simulink model "mchp_acim_dsPIC33A"  (R2025b)
settings: Solver=FixedStepDiscrete  StartTime=0.0  StopTime=25  FixedStep=Ts  RelTol=1e-3  EnableMultiTasking=on
values from neighbouring files (symbols this model uses):
  dataType = 'single'    [mchp_acim_foc_dsPIC33A_data.m]
  PWM_frequency = 20e3    (= 20000)    [mchp_acim_foc_dsPIC33A_data.m]
  PWM_frequency_mc = PWM_frequency    (= 20000)    [mchp_acim_foc_dsPIC33A_data.m]
  SpeedFilterCutoff = 40    [mchp_acim_foc_dsPIC33A_data.m]
  Ts = T_pwm    (= 5e-05)    [mchp_acim_foc_dsPIC33A_data.m]
  Ts_mc = T_pwm_mc    (= 5e-05)    [mchp_acim_foc_dsPIC33A_data.m]
  Ts_motor = T_pwm_mc    (= 5e-05)    [mchp_acim_foc_dsPIC33A_data.m]
  Ts_serialIn = 100e-3    (= 0.1)    [mchp_acim_foc_dsPIC33A_data.m]
undefined symbols (not defined in the file or in its folder): A0, A4, acim, ADC, appState, B0, C10, C11, C6, C7, C8, CS_param, D11, D12, DiscIntNeverNeededParam, estim_pll, estim_qei, inverter, Max, MaxPer, ms, NumBits1, NumBits2, P1, P17, P20, P39, P40, P41, P43, P44, P60, P61, PI_params_SI, Pin, PWM4_Trg1, Resol, s, target, us, VmaxPhase
libraries: simulink x47, MCHP_Blockset x24, mcbcontrolslib x5, mcbeeMathTransformLib x4, slpidlib x4, svdutilitieslib x1, autolibim x1, mcbplantlib x1
(part 5 of 6)

== system mchp_acim_dsPIC33A/MCHV-230VAC-1.5kW Development Board dsPIC33AK128MC106 MC DIM/Downsample x20 ==
  note: DownSample & Average by changing data scaling
  In1 : Inport
  Compare To Constant : simulink/Logic and Bit Operations/Compare To Constant  relop===  const=1  OutDataTypeStr=boolean
  Counter Limited : simulink/Sources/Counter Limited  uplimit=DownSample-1  tsamp=-1
  Data Type Duplicate : DataTypeDuplicate
  Data Type Propagation : simulink/Signal Attributes/Data Type Propagation  PropDataType=fixdt(1, 16)  IfRefDouble=double  IfRefSingle=single  IsSigned=IsSigned1 or IsSigned2  NumBitsBase=NumBits1+NumBits2  NumBitsMult=1  NumBitsAdd=0  NumBitsAllowFinal=-1  PropScaling=2^-10  ValuesUsedBestPrec=[5 -7]  SlopeBase=Slope1  SlopeMult=1  SlopeAdd=0  BiasBase=Bias1  BiasMult=1  BiasAdd=0
  Data Type Propagation1 : simulink/Signal Attributes/Data Type Propagation  PropDataType=fixdt(1, 16)  IfRefDouble=double  IfRefSingle=single  IsSigned=IsSigned1 or IsSigned2  NumBitsBase=NumBits1+NumBits2  NumBitsMult=1  NumBitsAdd=0  NumBitsAllowFinal=-1  PropScaling=2^-10  ValuesUsedBestPrec=[5 -7]  SlopeBase=PosRange1  SlopeMult=1  SlopeAdd=0  BiasBase=Bias1  BiasMult=1  BiasAdd=0
  Discrete-Time Integrator : DiscreteIntegrator  IntegratorMethod=Accumulation: Backward Euler  gainval=1  ExternalReset=sampled level  SampleTime=-1  OutDataTypeStr=Inherit: Inherit via back propagation  ICPrevOutput=DiscIntNeverNeededParam  ICPrevScaledInput=DiscIntNeverNeededParam
  Gain : Gain  Gain=1/DownSample  OutDataTypeStr=Inherit: Inherit via back propagation  RndMeth=Round
  Gain1 : Gain  Gain=1/DownSample  OutDataTypeStr=Inherit: Inherit via back propagation
  Rate Transition1 : RateTransition  OutPortSampleTimeOpt=Multiple of input port sample time  OutPortSampleTimeMultiple=DownSample  OutPortSampleTime=DownSample
  Rate Transition3 : RateTransition  OutPortSampleTimeOpt=Multiple of input port sample time  OutPortSampleTimeMultiple=DownSample  OutPortSampleTime=DownSample
  Terminator : Terminator
  Out1 : Outport  VectorParamsAs1DForOutWhenUnconnected=off
  wires:
  Rate Transition3/1 -> Gain1/1, Gain/1
  In1/1 -> Rate Transition1/1, Discrete-Time Integrator/1, Data Type Propagation/2, Data Type Propagation/1
  Compare To Constant/1 -> Discrete-Time Integrator/2
  Discrete-Time Integrator/1 -> Data Type Propagation/3, Rate Transition3/1
  Counter Limited/1 -> Compare To Constant/1
  Gain/1 -> Data Type Duplicate/2, Out1/1
  Rate Transition1/1 -> Data Type Propagation1/2, Data Type Propagation1/1, Data Type Duplicate/1
  Gain1/1 -> Terminator/1, Data Type Propagation1/3

== system mchp_acim_dsPIC33A/MCHV-230VAC-1.5kW Development Board dsPIC33AK128MC106 MC DIM/Downsample x20 _ ==
  note: DownSample & Average by changing data scaling
  In1 : Inport
  Compare To Constant : simulink/Logic and Bit Operations/Compare To Constant  relop===  const=1  OutDataTypeStr=boolean
  Counter Limited : simulink/Sources/Counter Limited  uplimit=DownSample-1  tsamp=-1
  Data Type Duplicate : DataTypeDuplicate
  Data Type Propagation : simulink/Signal Attributes/Data Type Propagation  PropDataType=fixdt(1, 16)  IfRefDouble=double  IfRefSingle=single  IsSigned=IsSigned1 or IsSigned2  NumBitsBase=NumBits1+NumBits2  NumBitsMult=1  NumBitsAdd=0  NumBitsAllowFinal=-1  PropScaling=2^-10  ValuesUsedBestPrec=[5 -7]  SlopeBase=Slope1  SlopeMult=1  SlopeAdd=0  BiasBase=Bias1  BiasMult=1  BiasAdd=0
  Data Type Propagation1 : simulink/Signal Attributes/Data Type Propagation  PropDataType=fixdt(1, 16)  IfRefDouble=double  IfRefSingle=single  IsSigned=IsSigned1 or IsSigned2  NumBitsBase=NumBits1+NumBits2  NumBitsMult=1  NumBitsAdd=0  NumBitsAllowFinal=-1  PropScaling=2^-10  ValuesUsedBestPrec=[5 -7]  SlopeBase=PosRange1  SlopeMult=1  SlopeAdd=0  BiasBase=Bias1  BiasMult=1  BiasAdd=0
  Discrete-Time Integrator : DiscreteIntegrator  IntegratorMethod=Accumulation: Backward Euler  gainval=1  ExternalReset=sampled level  SampleTime=-1  OutDataTypeStr=Inherit: Inherit via back propagation  ICPrevOutput=DiscIntNeverNeededParam  ICPrevScaledInput=DiscIntNeverNeededParam
  Gain : Gain  Gain=1/DownSample  OutDataTypeStr=Inherit: Inherit via back propagation  RndMeth=Round
  Gain1 : Gain  Gain=1/DownSample  OutDataTypeStr=Inherit: Inherit via back propagation
  Rate Transition1 : RateTransition  OutPortSampleTimeOpt=Multiple of input port sample time  OutPortSampleTimeMultiple=DownSample  OutPortSampleTime=DownSample
  Rate Transition3 : RateTransition  OutPortSampleTimeOpt=Multiple of input port sample time  OutPortSampleTimeMultiple=DownSample  OutPortSampleTime=DownSample
  Terminator : Terminator
  Out1 : Outport  VectorParamsAs1DForOutWhenUnconnected=off
  wires:
  Gain1/1 -> Data Type Propagation1/3, Terminator/1
  Rate Transition1/1 -> Data Type Duplicate/1, Data Type Propagation1/1, Data Type Propagation1/2
  Gain/1 -> Out1/1, Data Type Duplicate/2
  Counter Limited/1 -> Compare To Constant/1
  Discrete-Time Integrator/1 -> Rate Transition3/1, Data Type Propagation/3
  Compare To Constant/1 -> Discrete-Time Integrator/2
  In1/1 -> Data Type Propagation/1, Data Type Propagation/2, Discrete-Time Integrator/1, Rate Transition1/1
  Rate Transition3/1 -> Gain/1, Gain1/1

== system mchp_acim_dsPIC33A/MCHV-230VAC-1.5kW Development Board dsPIC33AK128MC106 MC DIM/MCHV-230VAC-1.5kW Development board webpage ==

== system mchp_acim_dsPIC33A/MCHV-230VAC-1.5kW Development Board dsPIC33AK128MC106 MC DIM/Timing Analysis ==
  note: CPU overload is 0 if no overload took place between two MCU Overload block execution.
      | Otherwise, bits field output code for TID(s) responsible for at least one overload.
  Downsample Averaged2 : Subsystem  mask{InputSampleTime=.0005, DownSample=200}
      mask prompts: InputSampleTime "Input sample time"; DownSample "DownSample Factor"
  Gain : Gain  Gain=5e-9/.0005 * 100  OutMin=0  OutMax=100  OutDataTypeStr=fixdt(0,16)  RndMeth=Simplest  SaturateOnIntegerOverflow=on
  MCU Load : MCHP_Blockset/Profiling/MCU Load  MCULoadPin_TXT=None  MCULoadMeasure=on  TIMER_Resolution_TXT="Resol: 0.005(us)  -  Max: 0.328(ms)"  MCHP_TIMER_REQUEST={MCU_Load}{MCU_Load}21:5:0:0:[]:32768;  MCHP_TIMER_RESULT=[2 65535 ]  MCHP_MASTERLINK=mchp_acim_dsPIC33A/MCHV-230VAC-1.5kW Development Board dsPIC33AK128MC106 MC DIM/Microchip Master  MCHP_COMPILED_INFO="CompiledSampleTime= [0.00050000000000000001041   0 ];CompiledInportDataTypes=[    ];CompiledInportDataWidth=[];"  Info="Timer 2:  Resol: 5(ns)  -  Max: 327.68(us)"  SampleTime=.0005
      settings: SourceProductName=MPLAB Device Blocks for Simulink
  MCU Overload : MCHP_Blockset/Profiling/MCU Overload  MCUOverloadBlockOutput=on  MCUOverLoadPin_TXT=None  MCHP_MASTERLINK=mchp_acim_dsPIC33A/MCHV-230VAC-1.5kW Development Board dsPIC33AK128MC106 MC DIM/Microchip Master  SampleTime=-1
      settings: SourceProductName=MPLAB Device Blocks for Simulink
  Overload : Constant  Value=65535  OutDataTypeStr=Inherit: Inherit via back propagation
  Rate Transition : RateTransition  Deterministic=off  OutPortSampleTime=.0005*200
  Switch : Switch  Criteria=u2 ~= 0  SaturateOnIntegerOverflow=off  InputSameDT=off
  CPU Load : Outport  Unit=%  SampleTime=.0005*200
  CPU Overload : Outport  Port=2
  wires:
  Rate Transition/1 -> Switch/2
  MCU Overload/1 -> Rate Transition/1, CPU Overload/1
  MCU Load/1 -> Downsample Averaged2/1(In1)
  Downsample Averaged2/1(Out1) -> Switch/3
  Switch/1 -> Gain/1
  Overload/1 -> Switch/1
  Gain/1 -> CPU Load/1

== system mchp_acim_dsPIC33A/Control algorithm/Application_Abstraction/Subsystem1 ==
  thetaMech_PU : Inport
  Enable : Inport  Port=2
  32-bit PU Angle integrator : Subsystem
  Add : Sum  OutDataTypeStr=single
  Data Type Conversion6 : DataTypeConversion  OutDataTypeStr=fixdt(1,16,15)  RndMeth=Nearest  SaturateOnIntegerOverflow=off
  Data Type Conversion7 : DataTypeConversion  OutDataTypeStr=fixdt(1,16,15)  SaturateOnIntegerOverflow=off  RndMeth=Floor  LockScale=on
  Delay One Step1 : Delay  DelayLength=1  InitialCondition=0  SampleTime=Ts_mc
  Delay One Step5 : Delay  DelayLength=1  InitialCondition=0  ExternalReset=Rising  SampleTime=Ts_mc
      settings: InputPortMap=u0,r5
  Ele_rad/s to mech_rpm : Gain  Gain=60/(2*pi*acim.p)  ParamDataTypeStr=single  OutDataTypeStr=single
  Gain1 : Gain  Gain=(2*estim_qei.zeta_TL/estim_qei.tau_TL)  ParamDataTypeStr=single  OutDataTypeStr=single
  Gain2 : Gain  Gain=Ts_mc*(1/(estim_qei.tau_TL)^2)  OutDataTypeStr=single
  Gain3 : Gain  Gain=acim.p  ParamDataTypeStr=single  OutDataTypeStr=Inherit: Same as input
  LPF : Subsystem
  Subtract5 : Sum  OutDataTypeStr=Inherit: Same as first input
  Sum3 : Sum  Inputs=|+-  OutDataTypeStr=fixdt(1,16,16)
  speed_mech_rpm : Outport
  wires:
  Sum3/1 -> Gain2/1, Gain1/1
  Subtract5/1 -> Delay One Step5/1, Add/1
  Gain2/1 -> Subtract5/1
  Enable/1 -> Delay One Step5/2
  Delay One Step5/1 -> Subtract5/2
  Gain1/1 -> Add/2
  LPF/1(Out) -> speed_mech_rpm/1
  Ele_rad/s to mech_rpm/1 -> LPF/1(In)
  32-bit PU Angle integrator/1(PU_angle_e) -> Delay One Step1/1
  Add/1 -> Ele_rad/s to mech_rpm/1, 32-bit PU Angle integrator/1(speed_ele_rad/s)
  thetaMech_PU/1 -> Data Type Conversion6/1
  Delay One Step1/1 -> Data Type Conversion7/1
  Gain3/1 -> Sum3/1
  Data Type Conversion7/1 -> Sum3/2
  Data Type Conversion6/1 -> Gain3/1

== system mchp_acim_dsPIC33A/Control algorithm/Command_Signals/Triggered Subsystem ==
  Trigger : TriggerPort  TriggerType=falling  VariantControl=Variant
  Delay : Delay  DelayLength=1  InitialCondition=0
  NOT : Logic  Operator=NOT  IconShape=distinctive  AllPortsSameDT=off  OutDataTypeStr=boolean
  RunCmd : Outport
  wires:
  NOT/1 -> RunCmd/1, Delay/1
  Delay/1 -> NOT/1

== system mchp_acim_dsPIC33A/Control algorithm/Data Monitoring/SerialInDrivers ==
  Compare To Constant : simulink/Logic and Bit Operations/Compare To Constant  relop=>=  const=8  OutDataTypeStr=boolean
  Data Type Conversion : DataTypeConversion  SaturateOnIntegerOverflow=off  RndMeth=Floor
  Triggered Subsystem : Subsystem  TreatAsAtomicUnit=on
  UART Rx : MCHP_Blockset/BUS UART/UART Rx  UART_REF=1  Flag_Out=on  Rx_Size_popup=User defined  Rx_Size=8  S_Rx_Size=8  Split=Read all received char  SplitChar=10  OutputDefault_popup=do nothing (end of output vector will be undefined)  OutputDefault=-1  ORDERING=None  SampleTime=Ts_serialIn  MCHP_MASTERLINK=mchp_acim_dsPIC33A/MCHV-230VAC-1.5kW Development Board dsPIC33AK128MC106 MC DIM/Microchip Master  MCHP_COMPILED_INFO="CompiledSampleTime= [0.10000000000000000555   0 ];CompiledInportDataTypes=[    ];CompiledInportDataWidth=[];"
      settings: SourceProductName=MPLAB Device Blocks for Simulink
  SCI_Data : Outport
  wires:
  Compare To Constant/1 -> Triggered Subsystem/Trigger
  UART Rx/1 -> Data Type Conversion/1
  UART Rx/2 -> Triggered Subsystem/1(In1)
  Triggered Subsystem/1(SCI_Data) -> SCI_Data/1
  Data Type Conversion/1 -> Compare To Constant/1

== system mchp_acim_dsPIC33A/Control algorithm/Data Monitoring/SerialOutDrivers ==
  SerialData : Inport
  codegen : Subsystem  VariantControl=(codegen)
  sim : Subsystem  VariantControl=(sim)

== system mchp_acim_dsPIC33A/Control algorithm/Data Monitoring/Subsystem ==
  DebugSel : Inport
  DebugData : Inport  Port=2
  1 : Constant  Value=[1 2]  OutDataTypeStr=uint16  SampleTime=-1
  2 : Constant  Value=[3 4]  OutDataTypeStr=uint16  SampleTime=-1
  3 : Constant  Value=[5 6]  OutDataTypeStr=uint16  SampleTime=-1
  4 : Constant  Value=[7 8]  OutDataTypeStr=uint16  SampleTime=-1
  5 : Constant  Value=[9 10]  OutDataTypeStr=uint16  SampleTime=-1
  6 : Constant  Value=[11 12]  OutDataTypeStr=uint16  SampleTime=-1
  Data_Conditioning_Tx : Subsystem  Variant=on
  Multiport Switch : MultiPortSwitch  Inputs=6  DiagnosticForDefault=None  OutDataTypeStr=uint16  RndMeth=Simplest  SaturateOnIntegerOverflow=off  InputSameDT=off
  Selector : Selector  InputPortWidth=12  IndexOptions=Index vector (port)  Indices=[1 3]  OutputSizes=1
  Debug_signal : Outport
  wires:
  4/1 -> Multiport Switch/5
  DebugData/1 -> Selector/1
  Data_Conditioning_Tx/1(Data_Log) -> Debug_signal/1
  5/1 -> Multiport Switch/6
  1/1 -> Multiport Switch/2
  3/1 -> Multiport Switch/4
  Multiport Switch/1 -> Selector/2
  2/1 -> Multiport Switch/3
  6/1 -> Multiport Switch/7
  Selector/1 -> Data_Conditioning_Tx/1(In1)
  DebugSel/1 -> Multiport Switch/1

== system mchp_acim_dsPIC33A/Control algorithm/Data Monitoring/Variant Subsystem ==
  SCI_Data : Inport
  Mode : Inport  Port=2
  Codegen : Subsystem  VariantControl=(codegen)
  Sim : Subsystem  VariantControl=(sim)
  ConfigAndCommand : Outport
  DebugSel : Outport  Port=2

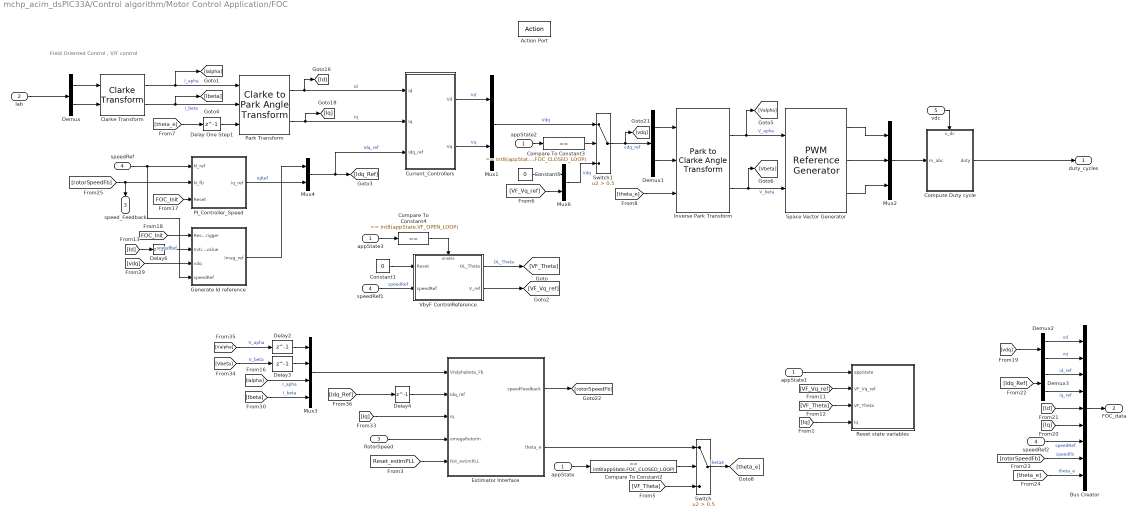
== system mchp_acim_dsPIC33A/Control algorithm/Motor Control Application/FOC ==
  note: Field Oriented Control , V/F control
  appState : Inport
  Iab : Inport  Port=2
  RotorSpeed : Inport  Port=3
  speedRef : Inport  Port=4
  vdc : Inport  Port=5
  Action Port : ActionPort  InitializeStates=reset  PropagateVarSize=During execution  ActionPortLabel=case [ VF_OPEN_LOOP FOC_CLOSED_LOOP ]:
  Bus Creator : BusCreator  Inputs=9
  Clarke Transform : mcbeeMathTransformLib/Clarke Transform  VariantControl=Variant2  PowerInvariant=off  UseWithEmbedded=on  PhaseInput=Two inputs
      settings: LibrarySourceBlock=mcbcontrolslib/Clarke Transform
  Compare To Constant2 : simulink/Logic and Bit Operations/Compare To Constant  relop===  const=int8(appState.FOC_CLOSED_LOOP)  OutDataTypeStr=boolean
  Compare To Constant3 : simulink/Logic and Bit Operations/Compare To Constant  relop===  const=int8(appState.FOC_CLOSED_LOOP)  OutDataTypeStr=boolean
  Compare To Constant4 : simulink/Logic and Bit Operations/Compare To Constant  relop===  const=int8(appState.VF_OPEN_LOOP)  OutDataTypeStr=boolean
  Compute Duty cycle : Subsystem
      settings: PortSchema="{\"entries\":[{\"content\":{\"sides\":[{\"content\":{\"connectorIds\":[\"In1\"]},\"type\":\"ConnectorPlacement.EquallySpacedRectSide\",\"uuid\":\"ac84263d-75b9-49d3-9a57-4d3cc97385b7\"},{\"content\":{\"connectorIds\":[\"Out1\"],\"side\":\"RIGHT\"},\"type\":\"ConnectorPlacement.EquallySpacedRectSide\",\"uuid\":\"0ce133fe-313b-45c1-86d5-76455f259936\"},{\"content\":{\"connectorIds\":[\"In2\"],\"side\":\"TOP\"},\"type\":\"ConnectorPlacement.EquallySpacedRectSide\",\"uuid\":\"39dacd62-df65-4cac-913f-002db890cfc1\"}]},\"type\":\"ConnectorPlacement.EquallySpacedConnector\",\"uuid\":\"58331c50-2548-46fe-a929-f01d574e6535\"}],\"packageUris\":[\"http://schema.mathworks.com/mf0/Connector/R2020b\"],\"version\":\"1.0\"}"
  Constant1 : Constant  Value=0  OutDataTypeStr=single  SampleTime=-1
  Constant5 : Constant  Value=0  OutDataTypeStr=single  SampleTime=-1
  Current_Controllers : Subsystem
  Delay One Step1 : Delay  DelayLength=1
  Delay2 : Delay  DelayLength=1
  Delay3 : Delay  DelayLength=1
  Delay4 : Delay  DelayLength=1  InitialCondition=[0.8, 0.05]
  Delay6 : Delay  DelayLength=1
  Demux{,1..3} (4 alike) : Demux  Outputs=2
  Estimator Interface : Subsystem
  Generate Id reference : Subsystem
  Inverse Park Transform : mcbeeMathTransformLib/Park to Clarke Angle Transform  AxisAlignment=D-axis  UseWithEmbedded=on  PhaseInput=Two inputs  ThetaInput=Electrical position  AngleInput=Radians  N_points=1024
      settings: LibrarySourceBlock=mcbcontrolslib/Inverse Park Transform
  Mux1 : Mux  Inputs=2
  Mux2 : Mux  Inputs=3
  Mux3 : Mux
  Mux4 : Mux  Inputs=2
  Mux6 : Mux  Inputs=2
  PI_Controller_Speed : Subsystem
  Park Transform : mcbeeMathTransformLib/Clarke to Park Angle Transform  AxisAlignment=D-axis  UseWithEmbedded=on  PhaseInput=Two inputs  ThetaInput=Electrical position  AngleInput=Radians  N_points=1024
      settings: LibrarySourceBlock=mcbcontrolslib/Park Transform
  Reset state variables : Subsystem
  Space Vector Generator : mcbcontrolslib/PWM Reference Generator  inSignal=Valphabeta  modType=SVM: space vector modulation
  Switch : Switch  Criteria=u2 > Threshold  Threshold=0.5  SaturateOnIntegerOverflow=off  InputSameDT=off
  Switch1 : Switch  Criteria=u2 > Threshold  Threshold=0.5  SaturateOnIntegerOverflow=off  InputSameDT=off
  VbyF ControlReference : Subsystem
  appState1 : InportShadow
  appState2 : InportShadow
  appState3 : InportShadow
  speedRef1 : InportShadow  Port=4
  speedRef2 : InportShadow  Port=4
  duty_cycles : Outport
  FOC_data : Outport  Port=2
  speed_Feedback : Outport  Port=3
  wires:
  Clarke Transform/2 -> [Ibeta], Park Transform/2  "I_beta"
  Demux/2 -> Clarke Transform/2
  Space Vector Generator/3 -> Mux2/3
  Park Transform/2 -> [Iq], Current_Controllers/2(Iq)  "Iq"
  Park Transform/1 -> [Id], Current_Controllers/1(Id)  "Id"
  Demux/1 -> Clarke Transform/1
  Inverse Park Transform/1 -> Space Vector Generator/1, [Valpha]  "V_apha"
  Clarke Transform/1 -> [Ialpha], Park Transform/1  "I_apha"
  Space Vector Generator/2 -> Mux2/2
  Inverse Park Transform/2 -> Space Vector Generator/2, [Vbeta]  "V_beta"
  Current_Controllers/1(Vd) -> Mux1/1  "Vd"
  Current_Controllers/2(Vq) -> Mux1/2  "Vq"
  Mux1/1 -> Switch1/1  "Vdq"
  Iab/1 -> Demux/1
  Bus Creator/1 -> FOC_data/1
  Demux1/1 -> Inverse Park Transform/1
  Demux1/2 -> Inverse Park Transform/2
  VbyF ControlReference/2(V_ref) -> [VF_Vq_ref]
  speedRef/1 -> Generate Id reference/4(speedRef), PI_Controller_Speed/1(N_ref)  "speedRef"
  VbyF ControlReference/1(OL_Theta) -> [VF_Theta]  "OL_Theta"
  Constant1/1 -> VbyF ControlReference/1(Reset)
  Generate Id reference/1(Imag_ref) -> Mux4/1
  PI_Controller_Speed/1(Iq_ref) -> Mux4/2  "IqRef"
  Mux4/1 -> [Idq_Ref], Current_Controllers/3(Idq_ref)  "Idq_ref"
  appState/1 -> Compare To Constant2/1
  [VF_Theta] -> Switch/3
  Compare To Constant2/1 -> Switch/2
  [VF_Vq_ref] -> Mux6/2
  Constant5/1 -> Mux6/1
  appState2/1 -> Compare To Constant3/1
  Compare To Constant3/1 -> Switch1/2
  Mux6/1 -> Switch1/3  "Vdq"
  Switch1/1 -> Demux1/1, [vdq]  "vdq_ref"
  [theta_e] -> Delay One Step1/1
  [theta_e] -> Inverse Park Transform/3
  speedRef1/1 -> VbyF ControlReference/2(speedRef)  "speedRef"
  [Id] -> Delay6/1
  Delay6/1 -> Generate Id reference/2(Initial_value)
  Space Vector Generator/1 -> Mux2/1
  [FOC_Init] -> PI_Controller_Speed/3(Reset)
  [FOC_Init] -> Generate Id reference/1(Reset_trigger)
  [vdq] -> Demux2/1
  [Idq_Ref] -> Demux3/1
  [Id] -> Bus Creator/5
  [Iq] -> Bus Creator/6
  [rotorSpeedFb] -> Bus Creator/8  "speedFb"
  [theta_e] -> Bus Creator/9  "theta_e"
  speedRef2/1 -> Bus Creator/7  "speedRef"
  [rotorSpeedFb] -> PI_Controller_Speed/2(N_fb), speed_Feedback/1
  Mux2/1 -> Compute Duty cycle/1(m_abc)
  Compute Duty cycle/1(duty) -> duty_cycles/1
  vdc/1 -> Compute Duty cycle/2(v_dc)
  [vdq] -> Generate Id reference/3(vdq)
  appState1/1 -> Reset state variables/1(appState)
  appState3/1 -> Compare To Constant4/1
  Compare To Constant4/1 -> VbyF ControlReference/Enable
  Mux3/1 -> Estimator Interface/1(VIalphabeta_Fb)
  [Idq_Ref] -> Delay4/1
  [Valpha] -> Delay2/1  "V_apha"
  Delay2/1 -> Mux3/1
  Delay4/1 -> Estimator Interface/2(Idq_ref)
  [Ibeta] -> Mux3/4  "I_beta"
  [Vbeta] -> Delay3/1  "V_beta"
  Delay3/1 -> Mux3/2
  [Ialpha] -> Mux3/3  "I_apha"
  [Iq] -> Estimator Interface/3(Iq)
  RotorSpeed/1 -> Estimator Interface/4(omegaRotorIn)
  Estimator Interface/1(speedFeedback) -> [rotorSpeedFb]
  Estimator Interface/2(theta_e) -> Switch/1
  Delay One Step1/1 -> Park Transform/3
  Switch/1 -> [theta_e]  "thetaE"
  [VF_Vq_ref] -> Reset state variables/2(VF_Vq_ref)
  [VF_Theta] -> Reset state variables/3(VF_Theta)
  [Iq] -> Reset state variables/4(Iq)
  Demux3/2 -> Bus Creator/4  "iq_ref"
  Demux3/1 -> Bus Creator/3  "id_ref"
  Demux2/2 -> Bus Creator/2  "vq"
  Demux2/1 -> Bus Creator/1  "vd"
  [Reset_estimPLL] -> Estimator Interface/5(Rst_estimPLL)

== system mchp_acim_dsPIC33A/Control algorithm/Motor Control Application/Switch Case Action Subsystem ==
  Action Port : ActionPort  ActionPortLabel=case [ INIT ]:
  Constant10 : Constant  Value=[0 0 0]  OutDataTypeStr=dataType  SampleTime=Ts_mc
  Duty_Cycles : Outport
  wires:
  Constant10/1 -> Duty_Cycles/1

== system mchp_acim_dsPIC33A/Control algorithm/Motor Control Application/Switch Case Action Subsystem1 ==
  Action Port : ActionPort  ActionPortLabel=case [ OFFSET_MEAS ]:
  Constant10 : Constant  Value=[0 0 0]  OutDataTypeStr=dataType  SampleTime=Ts_mc
  Duty_Cycles : Outport
  wires:
  Constant10/1 -> Duty_Cycles/1

== system mchp_acim_dsPIC33A/Control algorithm/Motor Control Application/Switch Case Action Subsystem6 ==
  Action Port : ActionPort  ActionPortLabel=case [ CMD_WAIT ]:
  Constant10 : Constant  Value=[0 0 0]  OutDataTypeStr=dataType  SampleTime=Ts_mc
  Duty_Cycles : Outport
  wires:
  Constant10/1 -> Duty_Cycles/1

== system mchp_acim_dsPIC33A/Control algorithm/Motor Control Application/Switch Case Action Subsystem8 ==
  Action Port : ActionPort  ActionPortLabel=case [ STOP ]:
  Constant10 : Constant  Value=[0 0 0]  OutDataTypeStr=dataType  SampleTime=Ts_mc
  Duty_Cycles : Outport
  wires:
  Constant10/1 -> Duty_Cycles/1

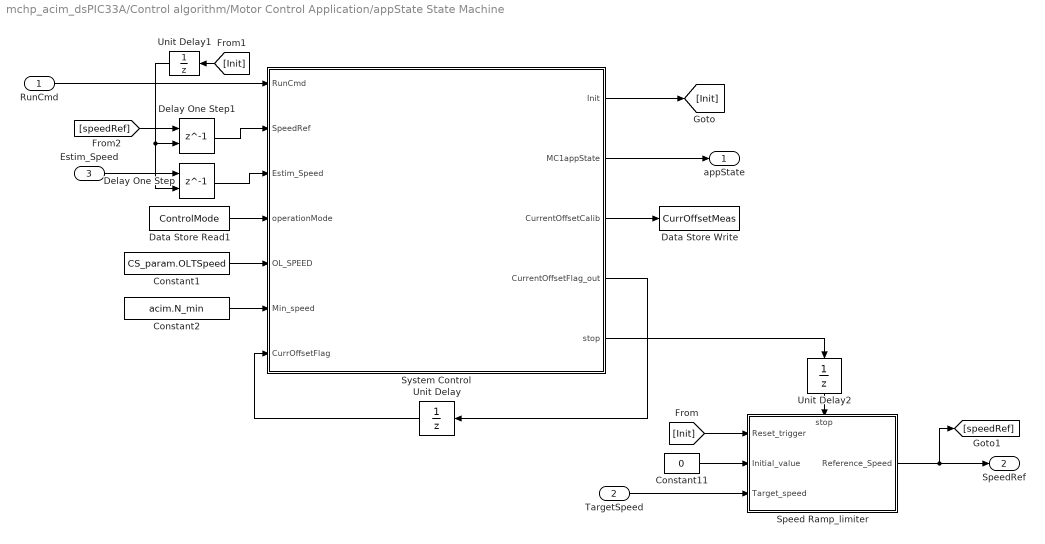
== system mchp_acim_dsPIC33A/Control algorithm/Motor Control Application/appState State Machine ==
  RunCmd : Inport
  TargetSpeed : Inport  Port=2
  Estim_Speed : Inport  Port=3
  Constant1 : Constant  Value=CS_param.OLTSpeed  OutDataTypeStr=single  SampleTime=-1
  Constant11 : Constant  Value=0  OutDataTypeStr=single  SampleTime=-1
  Constant2 : Constant  Value=acim.N_min  OutDataTypeStr=single  SampleTime=-1
  Data Store Read1 : DataStoreRead  DataStoreName=ControlMode  IndexOptions=Index vector (dialog)  Indices=1  OutputSizes=1
  Data Store Write : DataStoreWrite  DataStoreName=CurrOffsetMeas  IndexOptions=Index vector (dialog)  Indices=1  OutputSizes=1
  Delay One Step : Delay  DelayLength=1  ExternalReset=Rising
      settings: InputPortMap=u0,r5
  Delay One Step1 : Delay  DelayLength=1  ExternalReset=Rising
      settings: InputPortMap=u0,r5
  Speed Ramp_limiter : Subsystem
      settings: PortSchema="{\"entries\":[{\"content\":{\"sides\":[{\"content\":{\"connectorIds\":[\"In1\",\"In2\",\"In3\"]},\"type\":\"ConnectorPlacement.EquallySpacedRectSide\",\"uuid\":\"e8ad02be-694d-4221-8646-4c084b3944db\"},{\"content\":{\"connectorIds\":[\"Out1\"],\"side\":\"RIGHT\"},\"type\":\"ConnectorPlacement.EquallySpacedRectSide\",\"uuid\":\"a085ae95-de52-4e1d-a5b3-22bb50ad6f9b\"},{\"content\":{\"connectorIds\":[\"In4\"],\"side\":\"TOP\"},\"type\":\"ConnectorPlacement.EquallySpacedRectSide\",\"uuid\":\"9578737c-df7e-4f95-9460-5c8a62b1220e\"}]},\"type\":\"ConnectorPlacement.EquallySpacedConnector\",\"uuid\":\"d1810837-ee07-43de-beea-054fa145336d\"}],\"packageUris\":[\"http://schema.mathworks.com/mf0/Connector/R2020b\"],\"version\":\"1.0\"}"
  System Control : Stateflow chart  TreatAsAtomicUnit=on
      settings: PortSchema="{\"entries\":[{\"content\":{\"sides\":[{\"content\":{\"connectorIds\":[\"In1\",\"In2\",\"In5\",\"In3\",\"In4\",\"In6\",\"In7\"]},\"type\":\"ConnectorPlacement.EquallySpacedRectSide\",\"uuid\":\"55763e8d-7f73-4f84-bcf2-4b2b0f0a00bd\"},{\"content\":{\"connectorIds\":[\"Out2\",\"Out1\",\"Out3\",\"Out4\",\"Out5\"],\"side\":\"RIGHT\"},\"type\":\"ConnectorPlacement.EquallySpacedRectSide\",\"uuid\":\"fa80ef7b-287b-433f-8260-ff03a517800f\"},{\"content\":{\"side\":\"TOP\"},\"type\":\"ConnectorPlacement.EquallySpacedRectSide\",\"uuid\":\"8900c884-cbcc-4066-bc5f-6440d28e0400\"}]},\"type\":\"ConnectorPlacement.EquallySpacedConnector\",\"uuid\":\"d1ec0316-c890-471e-a041-a7780a4a6b79\"}],\"packageUris\":[\"http://schema.mathworks.com/mf0/Connector/R2020b\"],\"version\":\"1.0\"}"
  Unit Delay : UnitDelay  SampleTime=Ts_mc  HasFrameUpgradeWarning=on
  Unit Delay1 : UnitDelay  SampleTime=Ts_mc  HasFrameUpgradeWarning=on
  Unit Delay2 : UnitDelay  SampleTime=Ts_mc  HasFrameUpgradeWarning=on
  appState : Outport
  SpeedRef : Outport  Port=2
  wires:
  System Control/1(MC1appState) -> appState/1
  RunCmd/1 -> System Control/1(RunCmd)
  System Control/3(CurrentOffsetCalib) -> Data Store Write/1
  Speed Ramp_limiter/1(Reference_Speed) -> SpeedRef/1, [speedRef]
  System Control/4(CurrentOffsetFlag_out) -> Unit Delay/1
  Unit Delay/1 -> System Control/7(CurrOffsetFlag)
  Estim_Speed/1 -> Delay One Step/1
  Constant1/1 -> System Control/4(OL_SPEED)
  Delay One Step/1 -> System Control/5(Estim_Speed)
  Delay One Step1/1 -> System Control/2(SpeedRef)
  Unit Delay1/1 -> Delay One Step/2, Delay One Step1/2
  System Control/2(Init) -> [Init]
  Constant11/1 -> Speed Ramp_limiter/2(Initial_value)
  TargetSpeed/1 -> Speed Ramp_limiter/3(Target_speed)
  System Control/5(stop) -> Unit Delay2/1
  Unit Delay2/1 -> Speed Ramp_limiter/4(stop)
  Data Store Read1/1 -> System Control/3(operationMode)
  [Init] -> Unit Delay1/1
  [Init] -> Speed Ramp_limiter/1(Reset_trigger)
  [speedRef] -> Delay One Step1/1
  Constant2/1 -> System Control/6(Min_speed)

== system mchp_acim_dsPIC33A/Inverter and Motor model/Simulation/Load_Profile (Torque) ==
  Data Type Conversion : DataTypeConversion  OutDataTypeStr=single  SaturateOnIntegerOverflow=off  RndMeth=Floor
  IIR Filter : mcbcontrolslib/IIR Filter  VariantControl=Low Pass Filter  VariantSelect=Low-pass  FilterConstantInputType=Specify via dialog  Filter_constant=0.01  InitialOutput=Specify via dialog  InitialOutputValue=0  ExternalReset=none  advancedSettings=off  Ts=50e-6  cutOff_freq=32.1525
  Reversal : Step  Time=9
  Switch : Switch  Criteria=u2 > Threshold  SaturateOnIntegerOverflow=off  InputSameDT=off
  T_load : Step  Time=3  Before=0.05*acim.T_rated  After=0.3*acim.T_rated  SampleTime=Ts
  T_load1 : Step  Time=6  Before=0.3*acim.T_rated  After=-0.3*acim.T_rated  SampleTime=Ts
  Load_Trq : Outport  VectorParamsAs1DForOutWhenUnconnected=off
  wires:
  Switch/1 -> Data Type Conversion/1
  Data Type Conversion/1 -> IIR Filter/1
  IIR Filter/1 -> Load_Trq/1
  T_load1/1 -> Switch/1
  Reversal/1 -> Switch/2
  T_load/1 -> Switch/3

== system mchp_acim_dsPIC33A/Inverter and Motor model/Simulation/Motor and Inverter ==
  Vabc_In_PU : Inport
  Load : Inport  Port=2
  Bus Selector : BusSelector  OutputSignals=MtrMechPos
  Induction Motor : autolibim/Induction Motor  sim_type=Discrete  Ts=Ts_motor  port_config=Torque  P=acim.p  Zs=[acim.Rs, acim.Lls]  Zr=[acim.Rr, acim.Llr]  Lm=acim.Lm  mechanical=[acim.J, acim.B, 0]  theta_init=0  omega_init=0  RefBlkName='autolibim/Induction Motor'  aMode=5
      settings: LibrarySourceBlock=mcblib/Electrical Systems/Motors/Induction Motor
  Inverter : Subsystem
  RT1 : RateTransition  Deterministic=off  OutPortSampleTime=Ts_simulink
  RT3 : RateTransition  Deterministic=off  OutPortSampleTime=Ts_simulink
  Rate Transition : RateTransition  Integrity=off  OutPortSampleTime=Ts_motor
  Rate Transition1 : RateTransition  Integrity=off  OutPortSampleTime=Ts_motor
  Rate Transition2 : RateTransition  Deterministic=off  OutPortSampleTime=Ts
  Rate Transition3 : RateTransition  Deterministic=off  OutPortSampleTime=Ts
  Scope : Scope
      settings: ActiveDisplayYMinimum=-1  ActiveDisplayYMaximum=1  DataLoggingVariableName=ScopeData4
  Scope1 : Scope  NumInputPorts=2
      settings: ActiveDisplayYMinimum=-142.50303268432617  ActiveDisplayYMaximum=142.50303268432617  DataLoggingVariableName=ScopeData6
  Terminator1 : Terminator
  Iabc : Outport
  Theta : Outport  Port=2
  wires:
  Rate Transition3/1 -> Inverter/1(Duty_abc)
  Rate Transition2/1 -> Rate Transition1/1
  Bus Selector/1 -> Theta/1  "<MtrMechPos>"
  RT3/1 -> Bus Selector/1
  RT1/1 -> Iabc/1
  Vabc_In_PU/1 -> Rate Transition3/1
  Inverter/1(Vabc) -> Rate Transition/1
  Rate Transition1/1 -> Induction Motor/1
  Induction Motor/2 -> Scope1/2, RT1/1  "Iabc_motor"
  Rate Transition/1 -> Scope1/1, Induction Motor/2  "Vabc_motor"
  Load/1 -> Rate Transition2/1
  Induction Motor/1 -> RT3/1
  Induction Motor/3 -> Scope/1, Terminator1/1  "speed_plant_motor"

== system mchp_acim_dsPIC33A/Inverter and Motor model/Simulation/Sensor_Measurements ==
  note: Scaling
  note: Delays
  PhaseCurr : Inport
  pos : Inport  Port=2
  Bus Creator : BusCreator  Inputs=2
  Data Type Conversion2 : DataTypeConversion  OutDataTypeStr=single  RndMeth=Simplest  SaturateOnIntegerOverflow=off
  Data Type Conversion4 : DataTypeConversion  OutDataTypeStr=single  RndMeth=Simplest  SaturateOnIntegerOverflow=off
  Data Type Conversion7 : DataTypeConversion  OutDataTypeStr=single  RndMeth=Simplest  SaturateOnIntegerOverflow=off
  Delay1 : Delay  DelayLength=PI_params_SI.delay_Currents
  Delay2 : Delay  DelayLength=PI_params_SI.delay_Position
  Get_QEP_Counts : Gain  Gain=acim.QEPSlits*4/(2*pi)  OutDataTypeStr=int32  RndMeth=Simplest
  Selector : Selector  InputPortWidth=3  IndexOptions=Index vector (dialog)  Indices=[1 2]  OutputSizes=1
  Sim_fb : Outport  VectorParamsAs1DForOutWhenUnconnected=off
  wires:
  Delay1/1 -> Selector/1  "Iab_fb"
  Data Type Conversion4/1 -> Delay1/1
  Selector/1 -> Bus Creator/1  "Iab_plant_model"
  PhaseCurr/1 -> Data Type Conversion4/1
  Bus Creator/1 -> Sim_fb/1
  Data Type Conversion2/1 -> Delay2/1  "Theta_m_motor"
  Delay2/1 -> Get_QEP_Counts/1  "Theta_m"
  Get_QEP_Counts/1 -> Data Type Conversion7/1  "Theta_qep"
  pos/1 -> Data Type Conversion2/1
  Data Type Conversion7/1 -> Bus Creator/2  "position_count"

== system mchp_acim_dsPIC33A/MCHV-230VAC-1.5kW Development Board dsPIC33AK128MC106 MC DIM/Center & sign reversal/Downsample Averaged 2000 samples remove bias ==
  note: DownSample & Average by changing data scaling
  In1 : Inport
  Enable : EnablePort
  Compare To Constant : simulink/Logic and Bit Operations/Compare To Constant  relop===  const=1  OutDataTypeStr=boolean
  Counter Limited : simulink/Sources/Counter Limited  uplimit=DownSample-1  tsamp=-1
  Data Type Duplicate : DataTypeDuplicate
  Data Type Propagation : simulink/Signal Attributes/Data Type Propagation  PropDataType=fixdt(1, 16)  IfRefDouble=double  IfRefSingle=single  IsSigned=IsSigned1 or IsSigned2  NumBitsBase=NumBits1+NumBits2  NumBitsMult=1  NumBitsAdd=0  NumBitsAllowFinal=-1  PropScaling=2^-10  ValuesUsedBestPrec=[5 -7]  SlopeBase=Slope1  SlopeMult=1  SlopeAdd=0  BiasBase=Bias1  BiasMult=1  BiasAdd=0
  Data Type Propagation1 : simulink/Signal Attributes/Data Type Propagation  PropDataType=fixdt(1, 16)  IfRefDouble=double  IfRefSingle=single  IsSigned=IsSigned1 or IsSigned2  NumBitsBase=NumBits1+NumBits2  NumBitsMult=1  NumBitsAdd=0  NumBitsAllowFinal=-1  PropScaling=2^-10  ValuesUsedBestPrec=[5 -7]  SlopeBase=PosRange1  SlopeMult=1  SlopeAdd=0  BiasBase=Bias1  BiasMult=1  BiasAdd=0
  Discrete-Time Integrator : DiscreteIntegrator  IntegratorMethod=Accumulation: Backward Euler  gainval=1  ExternalReset=sampled level  SampleTime=-1  OutDataTypeStr=Inherit: Inherit via back propagation  ICPrevOutput=DiscIntNeverNeededParam  ICPrevScaledInput=DiscIntNeverNeededParam
  Gain : Gain  Gain=1/DownSample  OutDataTypeStr=uint16  RndMeth=Round
  Gain1 : Gain  Gain=1/DownSample  OutDataTypeStr=Inherit: Inherit via back propagation
  Gain2 : Gain  OutDataTypeStr=int32
  Rate Transition1 : RateTransition  OutPortSampleTimeOpt=Multiple of input port sample time  OutPortSampleTimeMultiple=DownSample  OutPortSampleTime=DownSample
  Rate Transition3 : RateTransition  OutPortSampleTimeOpt=Multiple of input port sample time  OutPortSampleTimeMultiple=DownSample  OutPortSampleTime=DownSample
  Terminator : Terminator
  Out1 : Outport  InitialOutput=[32768]  VectorParamsAs1DForOutWhenUnconnected=off
  wires:
  Gain1/1 -> Gain2/1, Data Type Propagation1/3  "Offset"
  Rate Transition1/1 -> Data Type Duplicate/1, Data Type Propagation1/1, Data Type Propagation1/2
  Gain/1 -> Terminator/1, Data Type Duplicate/2  "Offset_Value_Uint16"
  Counter Limited/1 -> Compare To Constant/1
  Discrete-Time Integrator/1 -> Rate Transition3/1, Data Type Propagation/3  "Intergrator_Out"
  Compare To Constant/1 -> Discrete-Time Integrator/2
  In1/1 -> Data Type Propagation/1, Data Type Propagation/2, Discrete-Time Integrator/1, Rate Transition1/1
  Rate Transition3/1 -> Gain/1, Gain1/1
  Gain2/1 -> Out1/1  "Offset_Value_int32"

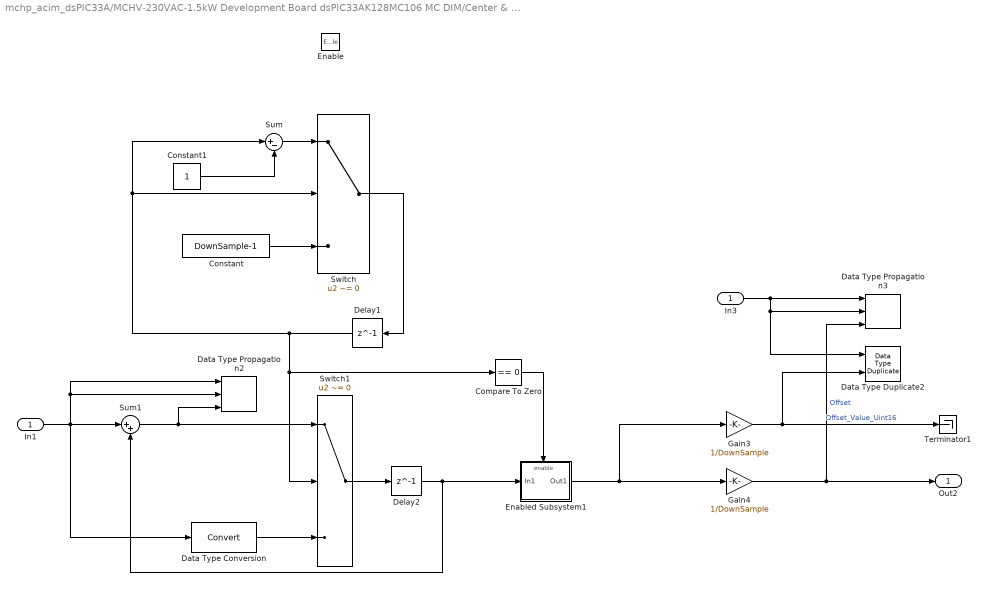
== system mchp_acim_dsPIC33A/MCHV-230VAC-1.5kW Development Board dsPIC33AK128MC106 MC DIM/Center & sign reversal1/Moving Average ==
  In1 : Inport
  Enable : EnablePort  ZeroCross=off
  Compare To Zero : simulink/Logic and Bit Operations/Compare To Zero  relop===  OutDataTypeStr=boolean
  Constant : Constant  Value=DownSample-1  OutDataTypeStr=uint16
  Constant1 : Constant  OutDataTypeStr=uint16
  Data Type Duplicate2 : DataTypeDuplicate
  Data Type Propagation2 : simulink/Signal Attributes/Data Type Propagation  PropDataType=fixdt(1, 16)  IfRefDouble=double  IfRefSingle=single  IsSigned=IsSigned1 or IsSigned2  NumBitsBase=NumBits1+NumBits2  NumBitsMult=1  NumBitsAdd=0  NumBitsAllowFinal=-1  PropScaling=2^-10  ValuesUsedBestPrec=[5 -7]  SlopeBase=Slope1  SlopeMult=1  SlopeAdd=0  BiasBase=Bias1  BiasMult=1  BiasAdd=0
  Data Type Propagation3 : simulink/Signal Attributes/Data Type Propagation  PropDataType=fixdt(1, 16)  IfRefDouble=double  IfRefSingle=single  IsSigned=IsSigned1 or IsSigned2  NumBitsBase=NumBits1+NumBits2  NumBitsMult=1  NumBitsAdd=0  NumBitsAllowFinal=-1  PropScaling=2^-10  ValuesUsedBestPrec=[5 -7]  SlopeBase=PosRange1  SlopeMult=1  SlopeAdd=0  BiasBase=Bias1  BiasMult=1  BiasAdd=0
  Data Type Conversion : DataTypeConversion  SaturateOnIntegerOverflow=off  RndMeth=Floor
  Delay1 : Delay  DelayLength=1  InitialCondition=0
  Delay2 : Delay  DelayLength=1  InitialCondition=[InitialValue * DownSample]
  Enabled Subsystem1 : Subsystem  TreatAsAtomicUnit=on
  Gain3 : Gain  Gain=1/DownSample  OutDataTypeStr=Inherit: Inherit via back propagation  RndMeth=Round
  Gain4 : Gain  Gain=1/DownSample  OutDataTypeStr=Inherit: Inherit via back propagation
  In3 : InportShadow
  Sum : Sum  Inputs=|+-  InputSameDT=on  OutDataTypeStr=Inherit: Same as first input
  Sum1 : Sum  Inputs=|++
  Switch : Switch  Criteria=u2 ~= 0  Threshold=DownSample-1  SaturateOnIntegerOverflow=off  InputSameDT=off
  Switch1 : Switch  Criteria=u2 ~= 0  Threshold=DownSample-1  SaturateOnIntegerOverflow=off
  Terminator1 : Terminator
  Out2 : Outport  InitialOutput=[InitialValue]  VectorParamsAs1DForOutWhenUnconnected=off
  wires:
  Switch/1 -> Delay1/1
  Sum/1 -> Switch/1
  Constant1/1 -> Sum/2
  Constant/1 -> Switch/3
  Delay1/1 -> Switch/2, Sum/1, Switch1/2, Compare To Zero/1
  Delay2/1 -> Sum1/2, Enabled Subsystem1/1(In1)
  In1/1 -> Data Type Conversion/1, Data Type Propagation2/2, Data Type Propagation2/1, Sum1/1
  Sum1/1 -> Data Type Propagation2/3, Switch1/1
  Switch1/1 -> Delay2/1
  Compare To Zero/1 -> Enabled Subsystem1/Enable
  Gain3/1 -> Data Type Duplicate2/2, Terminator1/1  "Offset_Value_Uint16"
  Enabled Subsystem1/1(Out1) -> Gain4/1, Gain3/1
  Gain4/1 -> Out2/1, Data Type Propagation3/3  "Offset"
  In3/1 -> Data Type Duplicate2/1, Data Type Propagation3/2, Data Type Propagation3/1
  Data Type Conversion/1 -> Switch1/3

== system mchp_acim_dsPIC33A/MCHV-230VAC-1.5kW Development Board dsPIC33AK128MC106 MC DIM/Timing Analysis/Downsample Averaged2 ==
  note: DownSample & Average by changing data scaling
  In1 : Inport
  Compare To Constant : simulink/Logic and Bit Operations/Compare To Constant  relop===  const=1  OutDataTypeStr=boolean
  Counter Limited : simulink/Sources/Counter Limited  uplimit=DownSample-1  tsamp=-1
  Data Type Duplicate : DataTypeDuplicate
  Data Type Propagation : simulink/Signal Attributes/Data Type Propagation  PropDataType=fixdt(1, 16)  IfRefDouble=double  IfRefSingle=single  IsSigned=IsSigned1 or IsSigned2  NumBitsBase=NumBits1+NumBits2  NumBitsMult=1  NumBitsAdd=0  NumBitsAllowFinal=-1  PropScaling=2^-10  ValuesUsedBestPrec=[5 -7]  SlopeBase=Slope1  SlopeMult=1  SlopeAdd=0  BiasBase=Bias1  BiasMult=1  BiasAdd=0
  Data Type Propagation1 : simulink/Signal Attributes/Data Type Propagation  PropDataType=fixdt(1, 16)  IfRefDouble=double  IfRefSingle=single  IsSigned=IsSigned1 or IsSigned2  NumBitsBase=NumBits1+NumBits2  NumBitsMult=1  NumBitsAdd=0  NumBitsAllowFinal=-1  PropScaling=2^-10  ValuesUsedBestPrec=[5 -7]  SlopeBase=PosRange1  SlopeMult=1  SlopeAdd=0  BiasBase=Bias1  BiasMult=1  BiasAdd=0
  Discrete-Time Integrator : DiscreteIntegrator  IntegratorMethod=Accumulation: Backward Euler  gainval=1  ExternalReset=sampled level  SampleTime=-1  OutDataTypeStr=Inherit: Inherit via back propagation  ICPrevOutput=DiscIntNeverNeededParam  ICPrevScaledInput=DiscIntNeverNeededParam
  Gain : Gain  Gain=1/DownSample  OutDataTypeStr=Inherit: Inherit via back propagation
  Gain1 : Gain  Gain=1/DownSample  OutDataTypeStr=Inherit: Inherit via back propagation
  Rate Transition1 : RateTransition  Deterministic=off  OutPortSampleTime=[InputSampleTime * DownSample]
  Rate Transition3 : RateTransition  OutPortSampleTime=[InputSampleTime * DownSample]
  Terminator : Terminator
  Out1 : Outport  VectorParamsAs1DForOutWhenUnconnected=off
  wires:
  Rate Transition3/1 -> Gain1/1, Gain/1
  In1/1 -> Discrete-Time Integrator/1, Rate Transition1/1, Data Type Propagation/2, Data Type Propagation/1
  Compare To Constant/1 -> Discrete-Time Integrator/2
  Discrete-Time Integrator/1 -> Data Type Propagation/3, Rate Transition3/1
  Counter Limited/1 -> Compare To Constant/1
  Gain/1 -> Data Type Duplicate/2, Out1/1
  Rate Transition1/1 -> Data Type Propagation1/2, Data Type Propagation1/1, Data Type Duplicate/1
  Gain1/1 -> Data Type Propagation1/3, Terminator/1

== system mchp_acim_dsPIC33A/Control algorithm/Application_Abstraction/Subsystem1/32-bit PU Angle integrator ==
  speed_ele_rad/s : Inport
  " " : Gain  Gain=Ts_mc  ParamDataTypeStr=single  OutDataTypeStr=single
  Data Type Conversion1 : DataTypeConversion  OutDataTypeStr=fixdt(1,32,31)  SaturateOnIntegerOverflow=off  RndMeth=Floor
  Data Type Conversion3 : DataTypeConversion  OutDataTypeStr=fixdt(1,16,15)  SaturateOnIntegerOverflow=off  RndMeth=Floor
  Delay One Step1 : Delay  DelayLength=1  InitialCondition=0  SampleTime=Ts_mc
  PU : Gain  Gain=1/pi  ParamDataTypeStr=single  OutDataTypeStr=single
  Subtract1 : Sum  OutDataTypeStr=fixdt(1,32,31)
  PU_angle_e : Outport
  wires:
  PU/1 -> Data Type Conversion1/1
  " "/1 -> PU/1
  Delay One Step1/1 -> Subtract1/2
  Data Type Conversion1/1 -> Subtract1/1
  Subtract1/1 -> Data Type Conversion3/1, Delay One Step1/1
  Data Type Conversion3/1 -> PU_angle_e/1
  speed_ele_rad/s/1 -> " "/1

== system mchp_acim_dsPIC33A/Control algorithm/Application_Abstraction/Subsystem1/LPF ==
  In : Inport
  Delay One Step : Delay  DelayLength=1  SampleTime=Ts_mc
  Gain : Gain  Gain=Ts_mc/((1/(2*pi*SpeedFilterCutoff))+Ts_mc)  ParamDataTypeStr=single  OutDataTypeStr=single
  Subtract : Sum  Inputs=+-
  Subtract1 : Sum  OutDataTypeStr=Inherit: Inherit via back propagation
  Out : Outport
  wires:
  In/1 -> Subtract/1
  Subtract1/1 -> Delay One Step/1, Out/1
  Delay One Step/1 -> Subtract1/2, Subtract/2
  Subtract/1 -> Gain/1
  Gain/1 -> Subtract1/1

== system mchp_acim_dsPIC33A/Control algorithm/Data Monitoring/SerialInDrivers/Triggered Subsystem ==
  In1 : Inport
  Trigger : TriggerPort  VariantControl=(inherit)
  SCI_Data : Outport
  wires:
  In1/1 -> SCI_Data/1

== system mchp_acim_dsPIC33A/Control algorithm/Data Monitoring/SerialOutDrivers/codegen ==
  SerialData : Inport
  SCI_Tx : Subsystem
  wires:
  SerialData/1 -> SCI_Tx/1(Data_Log)

== system mchp_acim_dsPIC33A/Control algorithm/Data Monitoring/SerialOutDrivers/sim ==
  SerialData : Inport
  Terminator : Terminator
  wires:
  SerialData/1 -> Terminator/1

== system mchp_acim_dsPIC33A/Control algorithm/Data Monitoring/Subsystem/Data_Conditioning_Tx ==
  In1 : Inport
  Data_Type_Fixed_Point : Subsystem  VariantControl=~isequal(dataType,'single')
  Data_Type_Float : Subsystem  VariantControl=isequal(dataType, 'single')
  Data_Log : Outport

== system mchp_acim_dsPIC33A/Control algorithm/Data Monitoring/Variant Subsystem/Codegen ==
  SCI_Data : Inport
  Mode : Inport  Port=2
  AND : Logic  IconShape=distinctive  AllPortsSameDT=off  OutDataTypeStr=boolean
  Bus Creator : BusCreator  Inputs=2
  Compare To Constant : simulink/Logic and Bit Operations/Compare To Constant  relop=>=  const=2  OutDataTypeStr=boolean
  Extract User inputs : Subsystem
  ConfigAndCommand : Outport
  DebugSel : Outport  Port=2
  wires:
  Bus Creator/1 -> ConfigAndCommand/1
  AND/1 -> Bus Creator/1  "Enable"
  SCI_Data/1 -> Extract User inputs/1(SCi_Data)
  Extract User inputs/3(DebugSel) -> DebugSel/1
  Mode/1 -> Compare To Constant/1
  Extract User inputs/2(SpeedRef) -> Bus Creator/2  "SpeedRef"
  Compare To Constant/1 -> AND/1
  Extract User inputs/1(Enable) -> AND/2

== system mchp_acim_dsPIC33A/Control algorithm/Data Monitoring/Variant Subsystem/Sim ==
  SCI_Data : Inport
  Mode : Inport  Port=2
  AND : Logic  IconShape=distinctive  AllPortsSameDT=off  OutDataTypeStr=boolean
  Bus Creator : BusCreator  Inputs=1
  Compare To Constant : simulink/Logic and Bit Operations/Compare To Constant  relop=>=  const=2  OutDataTypeStr=boolean
  DebugDataSel : Constant  OutDataTypeStr=uint8  SampleTime=-1
  Enable : Step  Time=9.5  Before=1  After=0  OutDataTypeStr=dataType
  Terminator : Terminator
  ConfigAndCommand : Outport
  DebugSel : Outport  Port=2
  wires:
  SCI_Data/1 -> Terminator/1
  Mode/1 -> Compare To Constant/1
  Compare To Constant/1 -> AND/2
  Bus Creator/1 -> ConfigAndCommand/1
  Enable/1 -> AND/1
  AND/1 -> Bus Creator/1  "Enable"
  DebugDataSel/1 -> DebugSel/1

== system mchp_acim_dsPIC33A/Control algorithm/Motor Control Application/FOC/Compute Duty cycle ==
  note: DC bus compensation
  note: Disable
  note: Enable
  m_abc : Inport
  v_dc : Inport  Port=2
  Constant2 : Constant  Value=inverter.V_dc  OutDataTypeStr=single  SampleTime=-1
  Constant4 : Constant  Value=0.5  OutDataTypeStr=dataType  SampleTime=-1
  Data Store Read : DataStoreRead  DataStoreName=DC_BusCompensation  IndexOptions=Index vector (dialog)  Indices=1  OutputSizes=1
  Gain : Gain  Gain=(sqrt(3))/2
  Math Reciprocal : Math  Operator=reciprocal  SignedPower=on
  Product : Product
  Saturation : Saturate  UpperLimit=0.88  LowerLimit=0.12
  Sum : Sum  Inputs=|++
  Switch : Switch  Criteria=u2 > Threshold  SaturateOnIntegerOverflow=off  InputSameDT=off
  duty : Outport
  wires:
  Constant4/1 -> Sum/2
  Sum/1 -> Saturation/1  "duty_cycles"
  Saturation/1 -> duty/1
  m_abc/1 -> Product/2
  Gain/1 -> Sum/1
  Math Reciprocal/1 -> Product/1
  Product/1 -> Gain/1
  v_dc/1 -> Switch/1
  Constant2/1 -> Switch/3
  Switch/1 -> Math Reciprocal/1
  Data Store Read/1 -> Switch/2

== system mchp_acim_dsPIC33A/Control algorithm/Motor Control Application/FOC/Current_Controllers ==
  Id : Inport
  Iq : Inport  Port=2
  Idq_ref : Inport  Port=3
  Demux : Demux  Outputs=2
  Dynamic Limit : Subsystem
  Mux : Mux
  PI_Controller_Id : Subsystem
  PI_Controller_Iq : Subsystem
  Terminator1 : Terminator
  Vd : Outport  VectorParamsAs1DForOutWhenUnconnected=off
  Vq : Outport  Port=2  VectorParamsAs1DForOutWhenUnconnected=off
  wires:
  Idq_ref/1 -> Demux/1
  Demux/2 -> PI_Controller_Iq/1(I_ref), Mux/3  "Iq_Ref"
  Demux/1 -> PI_Controller_Id/1(I_ref), Mux/1  "Id_Ref"
  Id/1 -> PI_Controller_Id/2(I_fb), Mux/2  "Id_fb"
  Iq/1 -> Mux/4, PI_Controller_Iq/2(I_fb)  "Iq_fb"
  Mux/1 -> Terminator1/1
  PI_Controller_Id/1(V_ref) -> Dynamic Limit/1(Vd), Vd/1
  Dynamic Limit/1(Vq_max) -> PI_Controller_Iq/3(Vq_max)
  PI_Controller_Iq/1(V_ref) -> Vq/1

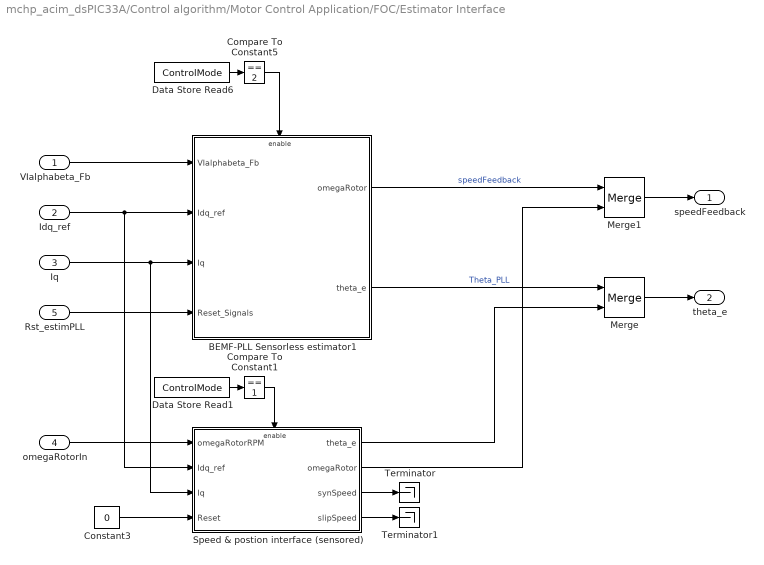
== system mchp_acim_dsPIC33A/Control algorithm/Motor Control Application/FOC/Estimator Interface ==
  VIalphabeta_Fb : Inport
  Idq_ref : Inport  Port=2
  Iq : Inport  Port=3
  omegaRotorIn : Inport  Port=4
  Rst_estimPLL : Inport  Port=5
  BEMF-PLL Sensorless estimator1 : Subsystem
  Compare To Constant1 : simulink/Logic and Bit Operations/Compare To Constant  relop===  const=1  OutDataTypeStr=boolean
  Compare To Constant5 : simulink/Logic and Bit Operations/Compare To Constant  relop===  const=2  OutDataTypeStr=boolean
  Constant3 : Constant  Value=0  OutDataTypeStr=single  SampleTime=-1
  Data Store Read1 : DataStoreRead  DataStoreName=ControlMode  IndexOptions=Index vector (dialog)  Indices=1  OutputSizes=1
  Data Store Read6 : DataStoreRead  DataStoreName=ControlMode  IndexOptions=Index vector (dialog)  Indices=1  OutputSizes=1
  Merge : Merge
  Merge1 : Merge
  Speed & postion interface (sensored) : Subsystem
  Terminator : Terminator
  Terminator1 : Terminator
  speedFeedback : Outport
  theta_e : Outport  Port=2
  wires:
  VIalphabeta_Fb/1 -> BEMF-PLL Sensorless estimator1/1(VIalphabeta_Fb)
  BEMF-PLL Sensorless estimator1/2(theta_e) -> Merge/1  "Theta_PLL"
  BEMF-PLL Sensorless estimator1/1(omegaRotor) -> Merge1/1  "speedFeedback"
  Iq/1 -> Speed & postion interface (sensored)/3(Iq), BEMF-PLL Sensorless estimator1/3(Iq)
  Speed & postion interface (sensored)/3(synSpeed) -> Terminator/1
  Speed & postion interface (sensored)/1(theta_e) -> Merge/2
  Speed & postion interface (sensored)/4(slipSpeed) -> Terminator1/1
  Idq_ref/1 -> Speed & postion interface (sensored)/2(Idq_ref), BEMF-PLL Sensorless estimator1/2(Idq_ref)
  Speed & postion interface (sensored)/2(omegaRotor) -> Merge1/2
  Merge1/1 -> speedFeedback/1
  Merge/1 -> theta_e/1
  omegaRotorIn/1 -> Speed & postion interface (sensored)/1(omegaRotorRPM)
  Constant3/1 -> Speed & postion interface (sensored)/4(Reset)
  Rst_estimPLL/1 -> BEMF-PLL Sensorless estimator1/4(Reset_Signals)
  Data Store Read6/1 -> Compare To Constant5/1
  Compare To Constant5/1 -> BEMF-PLL Sensorless estimator1/Enable
  Data Store Read1/1 -> Compare To Constant1/1
  Compare To Constant1/1 -> Speed & postion interface (sensored)/Enable

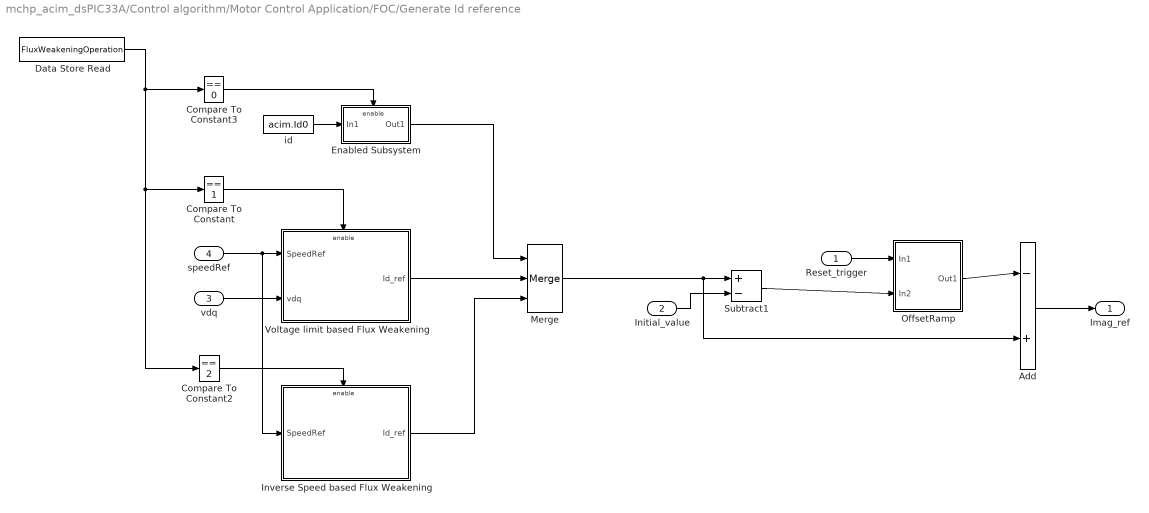
== system mchp_acim_dsPIC33A/Control algorithm/Motor Control Application/FOC/Generate Id reference ==
  Reset_trigger : Inport
  Initial_value : Inport  Port=2
  vdq : Inport  Port=3
  speedRef : Inport  Port=4
  Add : Sum  Inputs=-+
  Compare To Constant : simulink/Logic and Bit Operations/Compare To Constant  relop===  const=1  OutDataTypeStr=boolean
  Compare To Constant2 : simulink/Logic and Bit Operations/Compare To Constant  relop===  const=2  OutDataTypeStr=boolean
  Compare To Constant3 : simulink/Logic and Bit Operations/Compare To Constant  relop===  const=0  OutDataTypeStr=boolean
  Data Store Read : DataStoreRead  DataStoreName=FluxWeakeningOperation  IndexOptions=Index vector (dialog)  Indices=1  OutputSizes=1
  Enabled Subsystem : Subsystem  TreatAsAtomicUnit=on
  Inverse Speed based Flux Weakening : Subsystem
  Merge : Merge  Inputs=3
  OffsetRamp : Subsystem
  Subtract1 : Sum  Inputs=+-
  Voltage limit based Flux Weakening : Subsystem
  id : Constant  Value=acim.Id0  OutDataTypeStr=single  SampleTime=Ts_mc
  Imag_ref : Outport
  wires:
  Initial_value/1 -> Subtract1/2
  Merge/1 -> Add/2, Subtract1/1
  speedRef/1 -> Inverse Speed based Flux Weakening/1(SpeedRef), Voltage limit based Flux Weakening/1(SpeedRef)
  vdq/1 -> Voltage limit based Flux Weakening/2(vdq)
  Data Store Read/1 -> Compare To Constant2/1, Compare To Constant/1, Compare To Constant3/1
  Reset_trigger/1 -> OffsetRamp/1(In1)
  Subtract1/1 -> OffsetRamp/2(In2)
  OffsetRamp/1(Out1) -> Add/1
  Add/1 -> Imag_ref/1
  id/1 -> Enabled Subsystem/1(In1)
  Voltage limit based Flux Weakening/1(Id_ref) -> Merge/2
  Inverse Speed based Flux Weakening/1(Id_ref) -> Merge/3
  Compare To Constant/1 -> Voltage limit based Flux Weakening/Enable
  Compare To Constant2/1 -> Inverse Speed based Flux Weakening/Enable
  Enabled Subsystem/1(Out1) -> Merge/1
  Compare To Constant3/1 -> Enabled Subsystem/Enable
